simulink model "michal_model_1_5"  (R2019b)
settings: Solver=ode4  StartTime=0.0  StopTime=10.0  FixedStep=1e-2  RelTol=1e-3
values from neighbouring files (symbols this model uses):
  amplituda = 1    [s2.m]
  czestotliwosc = (2*pi*10)    (= 62.8318530718)    [s2.m]
  FinalValue = 0    [s2.m]
  InitialValue = 3    [s2.m]
  K = 1/(R*C)    (= 5)    [s2.m]
  SampleTime = 0    [s2.m]
  StepTime = 5    [s2.m]
  WPC = 4    [s2.m]
settings Model: Creator=resta  LastModifiedBy=resta

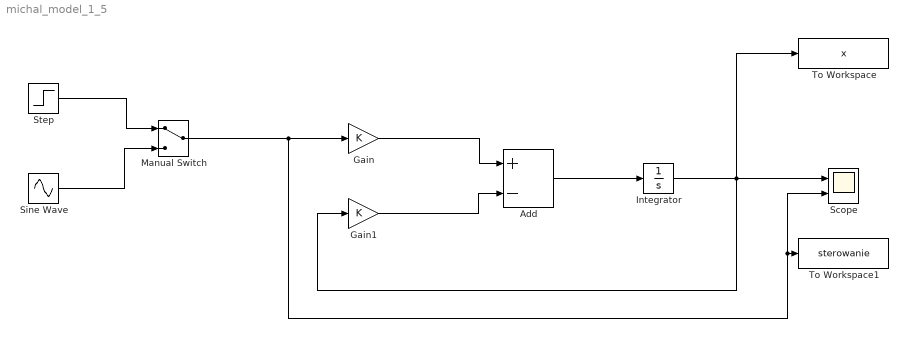
== system michal_model_1_5 ==
  Add : Sum  Inputs=+-
  Gain : Gain  Gain=K
  Gain1 : Gain  Gain=K
  Integrator : Integrator  InitialCondition=WPC
  Manual Switch : ManualSwitch
  Scope : Scope  NumInputPorts=2
  Sine Wave : Sin  Amplitude=amplituda  Frequency=czestotliwosc  SampleTime=0
  Step : Step  Time=StepTime  Before=InitialValue  After=FinalValue  SampleTime=SampleTime
  To Workspace : ToWorkspace  VariableName=x  SampleTime=-1
  To Workspace1 : ToWorkspace  VariableName=sterowanie  SampleTime=-1
  wires:
  Step/1 -> Manual Switch/1
  Sine Wave/1 -> Manual Switch/2
  Manual Switch/1 -> Scope/2, To Workspace1/1, Gain/1
  Gain/1 -> Add/1
  Gain1/1 -> Add/2
  Add/1 -> Integrator/1
  Integrator/1 -> Gain1/1, To Workspace/1, Scope/1
